simulink model "graphical_calc"  (R2018b)
settings: Solver=VariableStepAuto  StartTime=0.0  StopTime=10.0  RelTol=1e-3
settings Model: Creator=lenovo2  LastModifiedBy=lenovo2

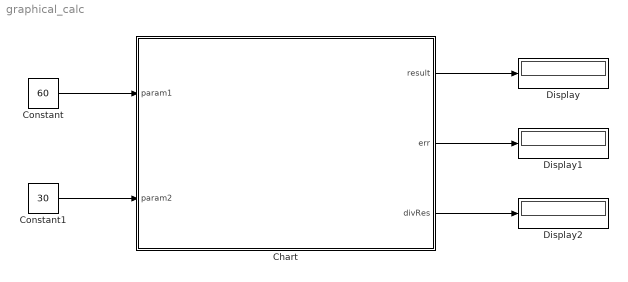
== system graphical_calc ==
  Chart : Stateflow chart  TreatAsAtomicUnit=on
  Constant : Constant  Value=60  OutDataTypeStr=uint8
  Constant1 : Constant  Value=30  OutDataTypeStr=uint8
  Display : Display
  Display1 : Display
  Display2 : Display
  wires:
  Chart/1(result) -> Display/1
  Constant/1 -> Chart/1(param1)
  Constant1/1 -> Chart/2(param2)
  Chart/2(err) -> Display1/1
  Chart/3(divRes) -> Display2/1

== stateflow chart graphical_calc/Chart ==
  state resultVal = add(n1,n2) [function]
    (default) -> (junction 6) : {resultVal= n1+n2;}
  state div(n1,n2) [function]
    (default) -> (junction 25) : % checkZero
    (junction 25) -> (junction 26) [order 1] : [n2==0]
    (junction 25) -> (junction 27) [order 2] : {divRes = n1/n2;}
    (junction 26) -> (junction 28) : {err = 0;}
    (junction 28) -> (junction 27)
    (junction 27) -> (junction 29)
  (default) -> (junction 1)
  (junction 1) -> (junction 3) : {result= add(param1,param2);
      | %after(2,sec);
      | div(param1,param2);
      | }
  data: n1 function_input; n2 function_input; resultVal function_output; n1 function_input; n2 function_input; param1 input uint8; param2 input uint8; result output uint8; err output uint8; divRes output uint8
